simulink model "AFST_DD"  (R2016b)
settings: configuration reference "CodeGenConfigSet" (kept outside this file)
values from neighbouring files (symbols this model uses):
  Air_bDtyOrUType_C = Calibration.Parameter    [init_AFST_DD.m]    (also in init_AFST_DD_SIL.m = Simulink.Parameter)
  Air_facPerCorTAFS_C = Calibration.Parameter    [init_AFST_DD.m]    (also in init_AFST_DD_SIL.m = Simulink.Parameter)
  Air_rDtyCycMaxTAFS_C = Calibration.Parameter    [init_AFST_DD.m]    (also in init_AFST_DD_SIL.m = Simulink.Parameter)
  Air_rDtyCycMinTAFS_C = Calibration.Parameter    [init_AFST_DD.m]    (also in init_AFST_DD_SIL.m = Simulink.Parameter)
  Air_swtOscSelTAFS_C = Calibration.Parameter    [init_AFST_DD.m]    (also in init_AFST_DD_SIL.m = Simulink.Parameter)
  Air_tiDtyCycHiTAFSDefDeb_C = Calibration.Parameter    [init_AFST_DD.m]    (also in init_AFST_DD_SIL.m = Simulink.Parameter)
  Air_tiDtyCycHiTAFSOKDeb_C = Calibration.Parameter    [init_AFST_DD.m]    (also in init_AFST_DD_SIL.m = Simulink.Parameter)
  Air_tiDtyCycLoTAFSDefDeb_C = Calibration.Parameter    [init_AFST_DD.m]    (also in init_AFST_DD_SIL.m = Simulink.Parameter)
  Air_tiDtyCycLoTAFSOKDeb_C = Calibration.Parameter    [init_AFST_DD.m]    (also in init_AFST_DD_SIL.m = Simulink.Parameter)
  Air_tiPerHiTAFSDefDeb_C = Calibration.Parameter    [init_AFST_DD.m]    (also in init_AFST_DD_SIL.m = Simulink.Parameter)
  Air_tiPerHiTAFSOKDeb_C = Calibration.Parameter    [init_AFST_DD.m]    (also in init_AFST_DD_SIL.m = Simulink.Parameter)
  Air_tiPerLoTAFSDefDeb_C = Calibration.Parameter    [init_AFST_DD.m]    (also in init_AFST_DD_SIL.m = Simulink.Parameter)
  Air_tiPerLoTAFSOKDeb_C = Calibration.Parameter    [init_AFST_DD.m]    (also in init_AFST_DD_SIL.m = Simulink.Parameter)
  Air_tiPerRefTAFS_C = Calibration.Parameter    [init_AFST_DD.m]    (also in init_AFST_DD_SIL.m = Simulink.Parameter)
  Air_tiRefSigPerMaxTAFS_C = Calibration.Parameter    [init_AFST_DD.m]    (also in init_AFST_DD_SIL.m = Simulink.Parameter)
  Air_tiRefSigPerMinTAFS_C = Calibration.Parameter    [init_AFST_DD.m]    (also in init_AFST_DD_SIL.m = Simulink.Parameter)
  Air_tiVoltHiTAFSDefDeb_C = Calibration.Parameter    [init_AFST_DD.m]    (also in init_AFST_DD_SIL.m = Simulink.Parameter)
  Air_tiVoltHiTAFSOKDeb_C = Calibration.Parameter    [init_AFST_DD.m]    (also in init_AFST_DD_SIL.m = Simulink.Parameter)
  Air_tiVoltLoTAFSDefDeb_C = Calibration.Parameter    [init_AFST_DD.m]    (also in init_AFST_DD_SIL.m = Simulink.Parameter)
  Air_tiVoltLoTAFSOKDeb_C = Calibration.Parameter    [init_AFST_DD.m]    (also in init_AFST_DD_SIL.m = Simulink.Parameter)
  Air_tTransfTAFS_CUR = Calibration.Parameter    [init_AFST_DD.m]    (also in init_AFST_DD_SIL.m = Simulink.Parameter)
  Air_tTransfTAFS_CURX = Calibration.Parameter    [init_AFST_DD.m]    (also in init_AFST_DD_SIL.m = Simulink.Parameter)
  Air_utTransfTAFS_CUR = Calibration.Parameter    [init_AFST_DD.m]    (also in init_AFST_DD_SIL.m = Simulink.Parameter)
  Air_utTransfTAFS_CURX = Calibration.Parameter    [init_AFST_DD.m]    (also in init_AFST_DD_SIL.m = Simulink.Parameter)
  Air_uVoltMaxTAFS_C = Calibration.Parameter    [init_AFST_DD.m]    (also in init_AFST_DD_SIL.m = Simulink.Parameter)
  Air_uVoltMinTAFS_C = Calibration.Parameter    [init_AFST_DD.m]    (also in init_AFST_DD_SIL.m = Simulink.Parameter)
undefined symbols (not defined in the file or in its folder): AFST_DD_DT, Switch_conv
libraries: CXLib x18
settings Model: Creator=Colin  LastModifiedBy=guanxiaoxing
settings ConfigSetRef: SourceLocation=Base Workspace

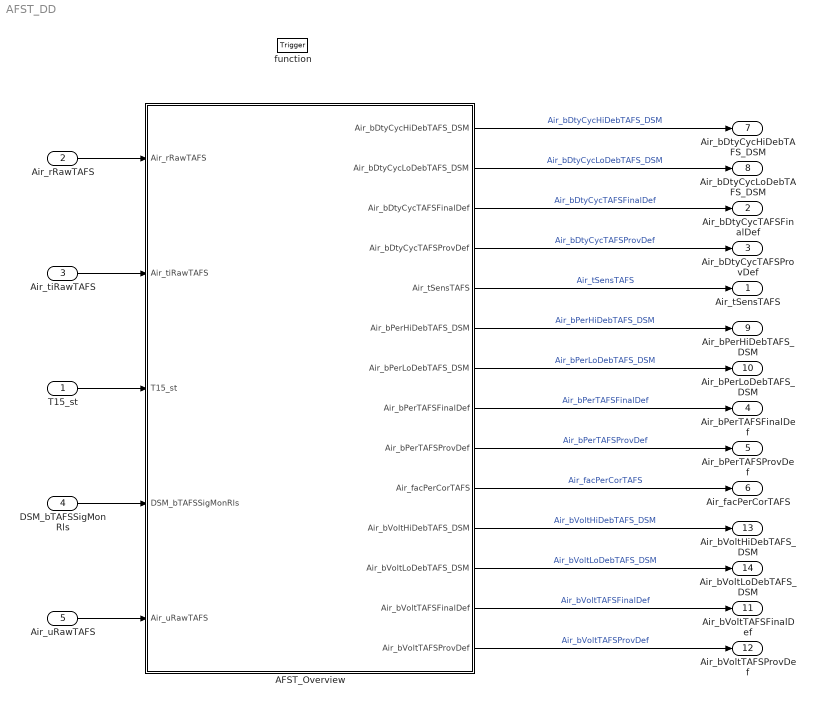
== system AFST_DD ==
  T15_st : Inport  Description=Terminal 15 status after debouncing  OutDataTypeStr=Enum: Switch_conv
  Air_rRawTAFS : Inport  Tag=%  Description=Duty cycle value of PWM signal from the temperature sensor at HFM position  Port=2  OutMin=0  OutMax=100  OutDataTypeStr=DutyCycle_rate
  Air_tiRawTAFS : Inport  Tag=ms  Description=Raw value of input time period of the temperature signal from HFM sensor  Port=3  OutMin=-107373  OutMax=107374  OutDataTypeStr=Time_Period_HFM6
  DSM_bTAFSSigMonRls : Inport  Description=fault flag of TAFS Signal Monitor  Port=4  OutMin=0  OutMax=1  OutDataTypeStr=boolean
  Air_uRawTAFS : Inport  Tag=mv  Description="Raw voltage value  from the temperature sensor at HFM position"  Port=5  OutMin=0  OutMax=5000  OutDataTypeStr=Ad_mv
  function : TriggerPort  TriggerType=function-call  VariantControl=Variant
  AFST_Overview : Subsystem
  Air_tSensTAFS : Outport  Tag=deg  Description=Sensed value of the air temperature at HFM position  OutMin=-200  OutMax=200  OutDataTypeStr=Temp_deg
  Air_bDtyCycTAFSFinalDef : Outport  Description=Fault flag of TAFS Duty Cycle Final fault  Port=2  OutMin=0  OutMax=1  OutDataTypeStr=boolean
  Air_bDtyCycTAFSProvDef : Outport  Description=Fault flag of TAFS Duty Cycle fault Proving  Port=3  OutMin=0  OutMax=1  OutDataTypeStr=boolean
  Air_bPerTAFSFinalDef : Outport  Description=Fault flag of TAFS Period Final fault  Port=4  OutMin=0  OutMax=1  OutDataTypeStr=boolean
  Air_bPerTAFSProvDef : Outport  Description=Fault flag of TAFS Period fault Proving  Port=5  OutMin=0  OutMax=1  OutDataTypeStr=boolean
  Air_facPerCorTAFS : Outport  Description=Period correction factor for air mass signal.  Port=6  OutMin=-4  OutMax=3.9999  OutDataTypeStr=Fact8192
  Air_bDtyCycHiDebTAFS_DSM : Outport  Description=Debounced fault of TAFS Duty Cycle High  Port=7  OutMin=0  OutMax=1  OutDataTypeStr=boolean
  Air_bDtyCycLoDebTAFS_DSM : Outport  Description=Debounced fault of TAFS Duty Cycle Low  Port=8  OutMin=0  OutMax=1  OutDataTypeStr=boolean
  Air_bPerHiDebTAFS_DSM : Outport  Description=Debounced fault of TAFS Period High  Port=9  OutMin=0  OutMax=1  OutDataTypeStr=boolean
  Air_bPerLoDebTAFS_DSM : Outport  Description=Debounced fault of TAFS Period Low  Port=10  OutMin=0  OutMax=1  OutDataTypeStr=boolean
  Air_bVoltTAFSFinalDef : Outport  Description=Fault flag of TAFS voltage Final fault  Port=11  OutMin=0  OutMax=1  OutDataTypeStr=boolean
  Air_bVoltTAFSProvDef : Outport  Description=Fault flag of TAFS voltage fault Proving  Port=12  OutMin=0  OutMax=1  OutDataTypeStr=boolean
  Air_bVoltHiDebTAFS_DSM : Outport  Description=Debounced fault of TAFS voltage High  Port=13  OutMin=0  OutMax=1  OutDataTypeStr=boolean
  Air_bVoltLoDebTAFS_DSM : Outport  Description="Debounced fault of TAFS  voltage Low"  Port=14  OutMin=0  OutMax=1  OutDataTypeStr=boolean
  wires:
  AFST_Overview/1(Air_bDtyCycHiDebTAFS_DSM) -> Air_bDtyCycHiDebTAFS_DSM/1  "Air_bDtyCycHiDebTAFS_DSM"
  AFST_Overview/3(Air_bDtyCycTAFSFinalDef) -> Air_bDtyCycTAFSFinalDef/1  "Air_bDtyCycTAFSFinalDef"
  AFST_Overview/4(Air_bDtyCycTAFSProvDef) -> Air_bDtyCycTAFSProvDef/1  "Air_bDtyCycTAFSProvDef"
  AFST_Overview/5(Air_tSensTAFS) -> Air_tSensTAFS/1  "Air_tSensTAFS"
  AFST_Overview/6(Air_bPerHiDebTAFS_DSM) -> Air_bPerHiDebTAFS_DSM/1  "Air_bPerHiDebTAFS_DSM"
  AFST_Overview/7(Air_bPerLoDebTAFS_DSM) -> Air_bPerLoDebTAFS_DSM/1  "Air_bPerLoDebTAFS_DSM"
  AFST_Overview/9(Air_bPerTAFSProvDef) -> Air_bPerTAFSProvDef/1  "Air_bPerTAFSProvDef"
  AFST_Overview/10(Air_facPerCorTAFS) -> Air_facPerCorTAFS/1  "Air_facPerCorTAFS"
  AFST_Overview/14(Air_bVoltTAFSProvDef) -> Air_bVoltTAFSProvDef/1  "Air_bVoltTAFSProvDef"
  AFST_Overview/11(Air_bVoltHiDebTAFS_DSM) -> Air_bVoltHiDebTAFS_DSM/1  "Air_bVoltHiDebTAFS_DSM"
  AFST_Overview/12(Air_bVoltLoDebTAFS_DSM) -> Air_bVoltLoDebTAFS_DSM/1  "Air_bVoltLoDebTAFS_DSM"
  AFST_Overview/2(Air_bDtyCycLoDebTAFS_DSM) -> Air_bDtyCycLoDebTAFS_DSM/1  "Air_bDtyCycLoDebTAFS_DSM"
  AFST_Overview/8(Air_bPerTAFSFinalDef) -> Air_bPerTAFSFinalDef/1  "Air_bPerTAFSFinalDef"
  AFST_Overview/13(Air_bVoltTAFSFinalDef) -> Air_bVoltTAFSFinalDef/1  "Air_bVoltTAFSFinalDef"
  Air_rRawTAFS/1 -> AFST_Overview/1(Air_rRawTAFS)
  Air_tiRawTAFS/1 -> AFST_Overview/2(Air_tiRawTAFS)
  T15_st/1 -> AFST_Overview/3(T15_st)
  DSM_bTAFSSigMonRls/1 -> AFST_Overview/4(DSM_bTAFSSigMonRls)
  Air_uRawTAFS/1 -> AFST_Overview/5(Air_uRawTAFS)

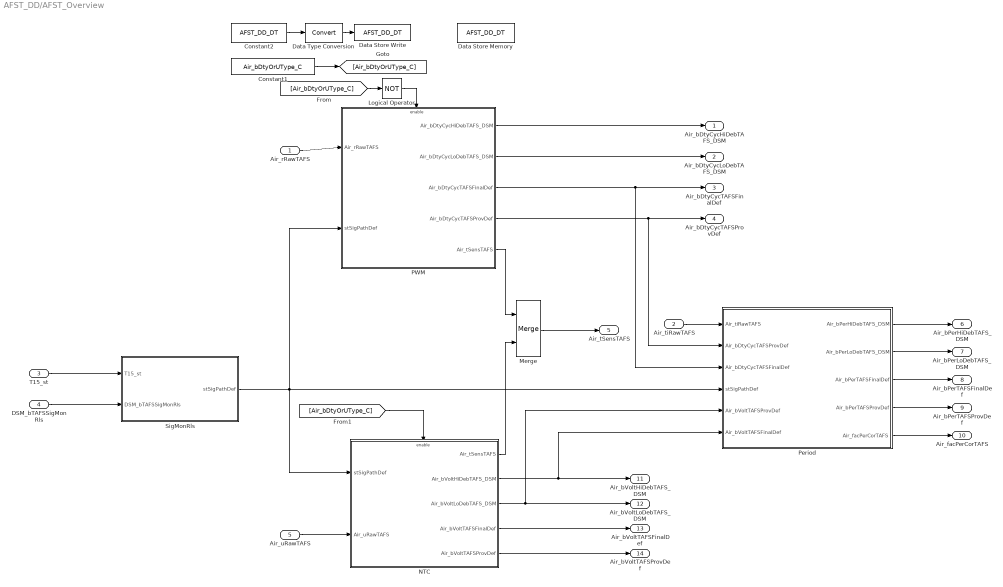
== system AFST_DD/AFST_Overview ==
  Air_rRawTAFS : Inport
  Air_tiRawTAFS : Inport  Port=2
  T15_st : Inport  Port=3
  DSM_bTAFSSigMonRls : Inport  Port=4
  Air_uRawTAFS : Inport  Port=5
  Constant1 : Constant  Value=Air_bDtyOrUType_C
  Constant2 : Constant  Value=AFST_DD_DT
  Data Store Memory : DataStoreMemory  DataStoreName=AFST_DD_DT  ReadBeforeWriteMsg=warning  WriteAfterWriteMsg=warning  WriteAfterReadMsg=warning  ShowAdditionalParam=off
  Data Store Write : DataStoreWrite  DataStoreName=AFST_DD_DT
  Data Type Conversion : DataTypeConversion
  Logical Operator : Logic  Operator=NOT  AllPortsSameDT=off  OutDataTypeStr=boolean
  Merge : Merge
  NTC : Subsystem
  PWM : Subsystem
  Period : Subsystem
  SigMonRls : Subsystem
  Air_bDtyCycHiDebTAFS_DSM : Outport
  Air_bDtyCycLoDebTAFS_DSM : Outport  Port=2
  Air_bDtyCycTAFSFinalDef : Outport  Port=3
  Air_bDtyCycTAFSProvDef : Outport  Port=4
  Air_tSensTAFS : Outport  Port=5
  Air_bPerHiDebTAFS_DSM : Outport  Port=6
  Air_bPerLoDebTAFS_DSM : Outport  Port=7
  Air_bPerTAFSFinalDef : Outport  Port=8
  Air_bPerTAFSProvDef : Outport  Port=9
  Air_facPerCorTAFS : Outport  Port=10
  Air_bVoltHiDebTAFS_DSM : Outport  Port=11
  Air_bVoltLoDebTAFS_DSM : Outport  Port=12
  Air_bVoltTAFSFinalDef : Outport  Port=13
  Air_bVoltTAFSProvDef : Outport  Port=14
  wires:
  NTC/3(Air_bVoltLoDebTAFS_DSM) -> Air_bVoltLoDebTAFS_DSM/1, Period/5(Air_bVoltTAFSProvDef)
  Period/4(Air_bPerTAFSProvDef) -> Air_bPerTAFSProvDef/1
  PWM/3(Air_bDtyCycTAFSFinalDef) -> Air_bDtyCycTAFSFinalDef/1, Period/3(Air_bDtyCycTAFSFinalDef)
  PWM/2(Air_bDtyCycLoDebTAFS_DSM) -> Air_bDtyCycLoDebTAFS_DSM/1
  NTC/4(Air_bVoltTAFSFinalDef) -> Air_bVoltTAFSFinalDef/1
  PWM/4(Air_bDtyCycTAFSProvDef) -> Air_bDtyCycTAFSProvDef/1, Period/2(Air_bDtyCycTAFSProvDef)
  DSM_bTAFSSigMonRls/1 -> SigMonRls/2(DSM_bTAFSSigMonRls)
  Constant2/1 -> Data Type Conversion/1
  Air_uRawTAFS/1 -> NTC/2(Air_uRawTAFS)
  Period/1(Air_bPerHiDebTAFS_DSM) -> Air_bPerHiDebTAFS_DSM/1
  NTC/5(Air_bVoltTAFSProvDef) -> Air_bVoltTAFSProvDef/1
  Merge/1 -> Air_tSensTAFS/1
  PWM/5(Air_tSensTAFS) -> Merge/1
  NTC/1(Air_tSensTAFS) -> Merge/2
  Air_rRawTAFS/1 -> PWM/1(Air_rRawTAFS)
  PWM/1(Air_bDtyCycHiDebTAFS_DSM) -> Air_bDtyCycHiDebTAFS_DSM/1
  [Air_bDtyOrUType_C] -> NTC/Enable
  Period/2(Air_bPerLoDebTAFS_DSM) -> Air_bPerLoDebTAFS_DSM/1
  Constant1/1 -> [Air_bDtyOrUType_C]
  T15_st/1 -> SigMonRls/1(T15_st)
  SigMonRls/1(stSigPathDef) -> PWM/2(stSigPathDef), Period/4(stSigPathDef), NTC/1(stSigPathDef)
  [Air_bDtyOrUType_C] -> Logical Operator/1
  Logical Operator/1 -> PWM/Enable
  Air_tiRawTAFS/1 -> Period/1(Air_tiRawTAFS)
  Data Type Conversion/1 -> Data Store Write/1
  NTC/2(Air_bVoltHiDebTAFS_DSM) -> Air_bVoltHiDebTAFS_DSM/1, Period/6(Air_bVoltTAFSFinalDef)
  Period/5(Air_facPerCorTAFS) -> Air_facPerCorTAFS/1
  Period/3(Air_bPerTAFSFinalDef) -> Air_bPerTAFSFinalDef/1

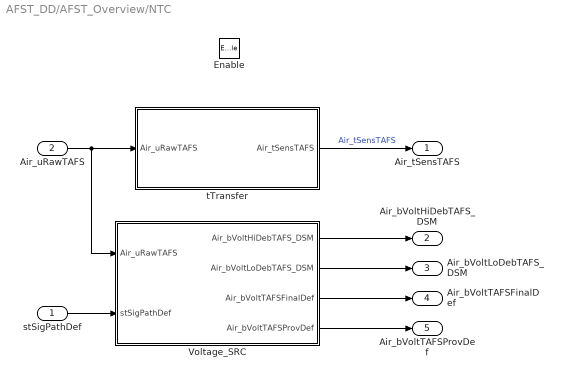
== system AFST_DD/AFST_Overview/NTC ==
  stSigPathDef : Inport
  Air_uRawTAFS : Inport  Port=2
  Enable : EnablePort
  Voltage_SRC : Subsystem
  tTransfer : Subsystem
  Air_tSensTAFS : Outport
  Air_bVoltHiDebTAFS_DSM : Outport  Port=2
  Air_bVoltLoDebTAFS_DSM : Outport  Port=3
  Air_bVoltTAFSFinalDef : Outport  Port=4
  Air_bVoltTAFSProvDef : Outport  Port=5
  wires:
  stSigPathDef/1 -> Voltage_SRC/2(stSigPathDef)
  Air_uRawTAFS/1 -> Voltage_SRC/1(Air_uRawTAFS), tTransfer/1(Air_uRawTAFS)
  tTransfer/1(Air_tSensTAFS) -> Air_tSensTAFS/1  "Air_tSensTAFS"
  Voltage_SRC/1(Air_bVoltHiDebTAFS_DSM) -> Air_bVoltHiDebTAFS_DSM/1
  Voltage_SRC/2(Air_bVoltLoDebTAFS_DSM) -> Air_bVoltLoDebTAFS_DSM/1
  Voltage_SRC/3(Air_bVoltTAFSFinalDef) -> Air_bVoltTAFSFinalDef/1
  Voltage_SRC/4(Air_bVoltTAFSProvDef) -> Air_bVoltTAFSProvDef/1

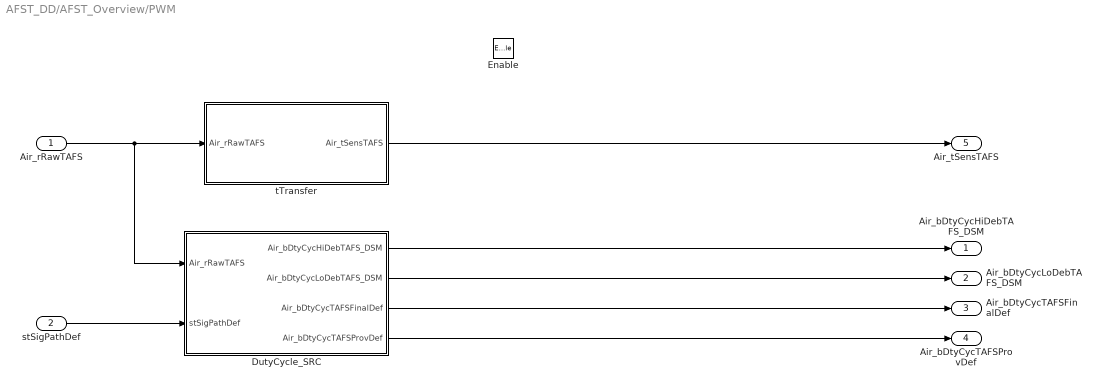
== system AFST_DD/AFST_Overview/PWM ==
  Air_rRawTAFS : Inport
  stSigPathDef : Inport  Port=2
  Enable : EnablePort
  "DutyCycle_SRC " : Subsystem
  tTransfer : Subsystem
  Air_bDtyCycHiDebTAFS_DSM : Outport
  Air_bDtyCycLoDebTAFS_DSM : Outport  Port=2
  Air_bDtyCycTAFSFinalDef : Outport  Port=3
  Air_bDtyCycTAFSProvDef : Outport  Port=4
  Air_tSensTAFS : Outport  Port=5
  wires:
  Air_rRawTAFS/1 -> tTransfer/1(Air_rRawTAFS), "DutyCycle_SRC "/1(Air_rRawTAFS)
  "DutyCycle_SRC "/3(Air_bDtyCycTAFSFinalDef) -> Air_bDtyCycTAFSFinalDef/1
  stSigPathDef/1 -> "DutyCycle_SRC "/2(stSigPathDef)
  "DutyCycle_SRC "/2(Air_bDtyCycLoDebTAFS_DSM) -> Air_bDtyCycLoDebTAFS_DSM/1
  "DutyCycle_SRC "/4(Air_bDtyCycTAFSProvDef) -> Air_bDtyCycTAFSProvDef/1
  "DutyCycle_SRC "/1(Air_bDtyCycHiDebTAFS_DSM) -> Air_bDtyCycHiDebTAFS_DSM/1
  tTransfer/1(Air_tSensTAFS) -> Air_tSensTAFS/1

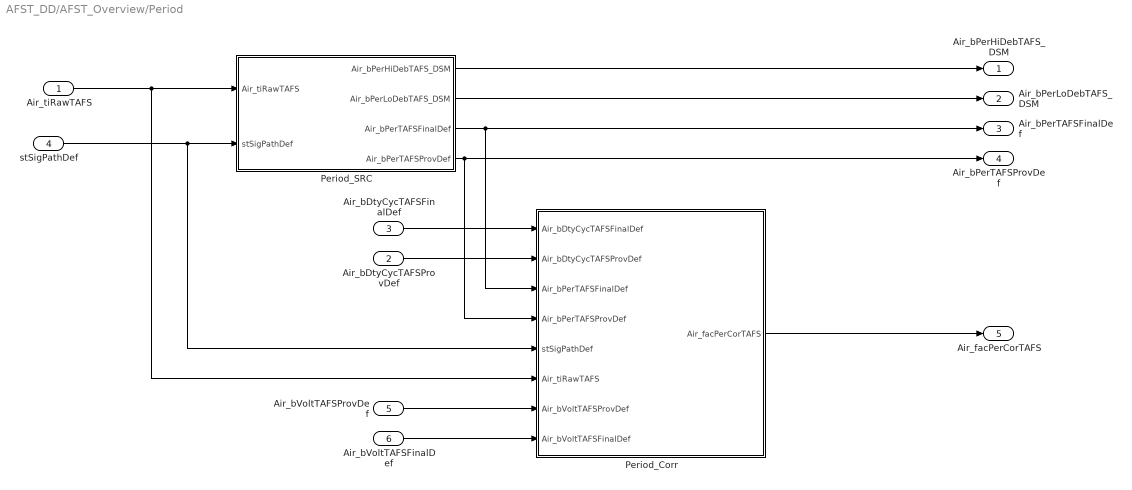
== system AFST_DD/AFST_Overview/Period ==
  Air_tiRawTAFS : Inport
  Air_bDtyCycTAFSProvDef : Inport  Port=2
  Air_bDtyCycTAFSFinalDef : Inport  Port=3
  stSigPathDef : Inport  Port=4
  Air_bVoltTAFSProvDef : Inport  Port=5
  Air_bVoltTAFSFinalDef : Inport  Port=6
  Period_Corr : Subsystem
  Period_SRC : Subsystem
  Air_bPerHiDebTAFS_DSM : Outport
  Air_bPerLoDebTAFS_DSM : Outport  Port=2
  Air_bPerTAFSFinalDef : Outport  Port=3
  Air_bPerTAFSProvDef : Outport  Port=4
  Air_facPerCorTAFS : Outport  Port=5
  wires:
  Air_tiRawTAFS/1 -> Period_SRC/1(Air_tiRawTAFS), Period_Corr/6(Air_tiRawTAFS)
  Period_SRC/4(Air_bPerTAFSProvDef) -> Air_bPerTAFSProvDef/1, Period_Corr/4(Air_bPerTAFSProvDef)
  Period_Corr/1(Air_facPerCorTAFS) -> Air_facPerCorTAFS/1
  Period_SRC/3(Air_bPerTAFSFinalDef) -> Air_bPerTAFSFinalDef/1, Period_Corr/3(Air_bPerTAFSFinalDef)
  Period_SRC/2(Air_bPerLoDebTAFS_DSM) -> Air_bPerLoDebTAFS_DSM/1
  Period_SRC/1(Air_bPerHiDebTAFS_DSM) -> Air_bPerHiDebTAFS_DSM/1
  Air_bDtyCycTAFSProvDef/1 -> Period_Corr/2(Air_bDtyCycTAFSProvDef)
  Air_bDtyCycTAFSFinalDef/1 -> Period_Corr/1(Air_bDtyCycTAFSFinalDef)
  stSigPathDef/1 -> Period_SRC/2(stSigPathDef), Period_Corr/5(stSigPathDef)
  Air_bVoltTAFSFinalDef/1 -> Period_Corr/8(Air_bVoltTAFSFinalDef)
  Air_bVoltTAFSProvDef/1 -> Period_Corr/7(Air_bVoltTAFSProvDef)

== system AFST_DD/AFST_Overview/SigMonRls ==
  T15_st : Inport
  DSM_bTAFSSigMonRls : Inport  Port=2
  Constant : Constant  Value=Switch_conv.ON
  Logical Operator : Logic  AllPortsSameDT=off  OutDataTypeStr=boolean
  Relational Operator : RelationalOperator  Operator===  OutDataTypeStr=boolean  RndMeth=Simplest
  stSigPathDef : Outport
  wires:
  T15_st/1 -> Relational Operator/1
  Logical Operator/1 -> stSigPathDef/1
  Relational Operator/1 -> Logical Operator/1
  DSM_bTAFSSigMonRls/1 -> Logical Operator/2
  Constant/1 -> Relational Operator/2

== system AFST_DD/AFST_Overview/NTC/Voltage_SRC ==
  Air_uRawTAFS : Inport
  stSigPathDef : Inport  Port=2
  FinalDef : Subsystem
  ProvDef : Subsystem
  SRCHi : Subsystem
  SRCLo : Subsystem
  Air_bVoltHiDebTAFS_DSM : Outport
  Air_bVoltLoDebTAFS_DSM : Outport  Port=2
  Air_bVoltTAFSFinalDef : Outport  Port=3
  Air_bVoltTAFSProvDef : Outport  Port=4
  wires:
  Air_uRawTAFS/1 -> SRCLo/1(Air_uRawTAFS), SRCHi/1(Air_uRawTAFS)
  SRCHi/1(Air_bVoltHiDebTAFS_DSM) -> FinalDef/1(Air_bVoltHiDebTAFS_DSM), Air_bVoltHiDebTAFS_DSM/1
  SRCLo/1(Air_bVoltLoDebTAFS_DSM) -> Air_bVoltLoDebTAFS_DSM/1, FinalDef/2(Air_bVoltLoDebTAFS_DSM)
  stSigPathDef/1 -> SRCHi/2(stSigPathDef), SRCLo/2(stSigPathDef), FinalDef/3(stSigPathDef)
  SRCLo/2(bVoltLo) -> ProvDef/3(bVoltLo)
  SRCHi/2(bVoltHi) -> ProvDef/2(bVoltHi)
  FinalDef/1(Air_bVoltTAFSFinalDef) -> Air_bVoltTAFSFinalDef/1, ProvDef/1(Air_bVoltTAFSFinalDef)
  ProvDef/1(Air_bVoltTAFSProvDef) -> Air_bVoltTAFSProvDef/1

== system AFST_DD/AFST_Overview/NTC/tTransfer ==
  Air_uRawTAFS : Inport
  Air_utTransfTAFS_CUR : Lookup_n-D  NumberOfTableDimensions=1  BreakpointsForDimension1=Air_utTransfTAFS_CURX  BreakpointsForDimension2=[1:3]  IndexSearchMethod=Linear search  BeginIndexSearchUsingPreviousIndexResult=on  Table=Air_utTransfTAFS_CUR  TableDataTypeStr=Inherit: Inherit from 'Table data'  ExtrapMethod=Clip  InternalRulePriority=Speed  OutDataTypeStr=Inherit: Inherit from 'Table data'  RndMeth=Simplest  InputSameDT=on
  Air_tSensTAFS : Outport
  wires:
  Air_uRawTAFS/1 -> Air_utTransfTAFS_CUR/1
  Air_utTransfTAFS_CUR/1 -> Air_tSensTAFS/1

== system AFST_DD/AFST_Overview/PWM/DutyCycle_SRC  ==
  Air_rRawTAFS : Inport
  stSigPathDef : Inport  Port=2
  FinalDef : Subsystem
  ProvDef : Subsystem
  SRCHi : Subsystem
  SRCLo : Subsystem
  Air_bDtyCycHiDebTAFS_DSM : Outport
  Air_bDtyCycLoDebTAFS_DSM : Outport  Port=2
  Air_bDtyCycTAFSFinalDef : Outport  Port=3
  Air_bDtyCycTAFSProvDef : Outport  Port=4
  wires:
  Air_rRawTAFS/1 -> SRCLo/1(Air_rRawTAFS), SRCHi/1(Air_rRawTAFS)
  SRCHi/1(Air_bDtyCycHiDebTAFS_DSM) -> FinalDef/1(Air_bDtyCycHiDebTAFS_DSM), Air_bDtyCycHiDebTAFS_DSM/1
  SRCLo/1(Air_bDtyCycLoDebTAFS_DSM) -> Air_bDtyCycLoDebTAFS_DSM/1, FinalDef/2(Air_bDtyCycLoDebTAFS_DSM)
  stSigPathDef/1 -> SRCHi/2(stSigPathDef), SRCLo/2(stSigPathDef), FinalDef/3(stSigPathDef)
  SRCLo/2(bDtyCycLo) -> ProvDef/3(bDtyCycLo)
  SRCHi/2(bDtyCycHi) -> ProvDef/2(bDtyCycHi)
  FinalDef/1(Air_bDtyCycTAFSFinalDef) -> Air_bDtyCycTAFSFinalDef/1, ProvDef/1(Air_bDtyCycTAFSFinalDef)
  ProvDef/1(Air_bDtyCycTAFSProvDef) -> Air_bDtyCycTAFSProvDef/1

== system AFST_DD/AFST_Overview/PWM/tTransfer ==
  Air_rRawTAFS : Inport
  Air_tTransfTAFS_CUR : Lookup_n-D  NumberOfTableDimensions=1  BreakpointsForDimension1=Air_tTransfTAFS_CURX  BreakpointsForDimension2=[1:3]  IndexSearchMethod=Linear search  BeginIndexSearchUsingPreviousIndexResult=on  Table=Air_tTransfTAFS_CUR  TableDataTypeStr=Inherit: Inherit from 'Table data'  ExtrapMethod=Clip  InternalRulePriority=Speed  OutDataTypeStr=Inherit: Inherit from 'Table data'  RndMeth=Simplest  InputSameDT=on
  Air_tSensTAFS : Outport
  wires:
  Air_rRawTAFS/1 -> Air_tTransfTAFS_CUR/1
  Air_tTransfTAFS_CUR/1 -> Air_tSensTAFS/1

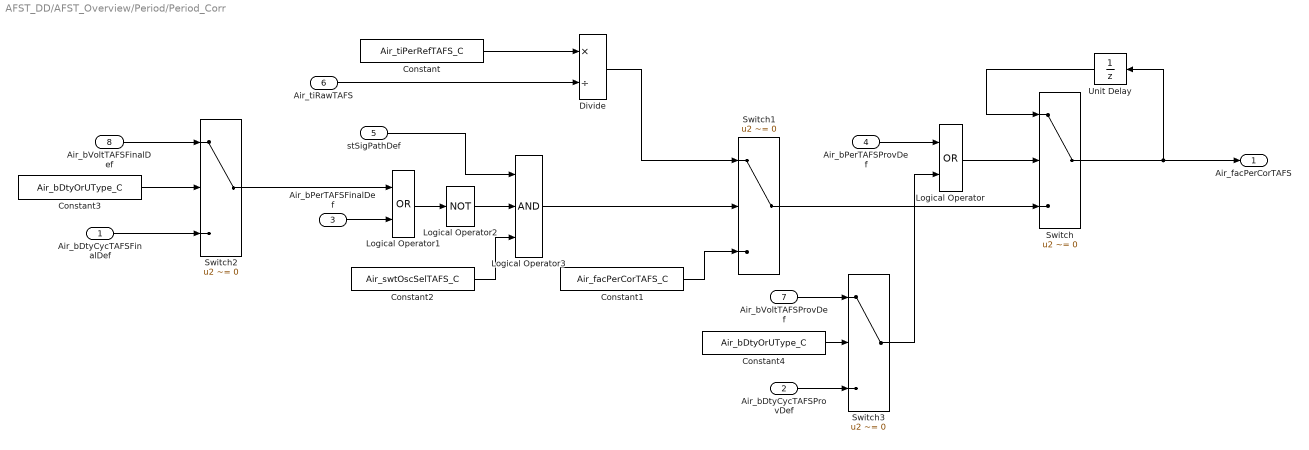
== system AFST_DD/AFST_Overview/Period/Period_Corr ==
  Air_bDtyCycTAFSFinalDef : Inport
  Air_bDtyCycTAFSProvDef : Inport  Port=2
  Air_bPerTAFSFinalDef : Inport  Port=3
  Air_bPerTAFSProvDef : Inport  Port=4
  stSigPathDef : Inport  Port=5
  Air_tiRawTAFS : Inport  Port=6
  Air_bVoltTAFSProvDef : Inport  Port=7
  Air_bVoltTAFSFinalDef : Inport  Port=8
  Constant : Constant  Value=Air_tiPerRefTAFS_C
  Constant1 : Constant  Value=Air_facPerCorTAFS_C
  Constant2 : Constant  Value=Air_swtOscSelTAFS_C
  Constant3 : Constant  Value=Air_bDtyOrUType_C
  Constant4 : Constant  Value=Air_bDtyOrUType_C
  Divide : Product  Inputs=*/  OutDataTypeStr=Inherit: Inherit via back propagation
  Logical Operator : Logic  Operator=OR  AllPortsSameDT=off  OutDataTypeStr=boolean
  Logical Operator1 : Logic  Operator=OR  AllPortsSameDT=off  OutDataTypeStr=boolean
  Logical Operator2 : Logic  Operator=NOT  AllPortsSameDT=off  OutDataTypeStr=boolean
  Logical Operator3 : Logic  Inputs=3  AllPortsSameDT=off  OutDataTypeStr=boolean
  Switch : Switch  Criteria=u2 ~= 0  OutDataTypeStr=Inherit: Inherit via back propagation
  Switch1 : Switch  Criteria=u2 ~= 0  OutDataTypeStr=Inherit: Inherit via back propagation  InputSameDT=on
  Switch2 : Switch  Criteria=u2 ~= 0  OutDataTypeStr=Inherit: Inherit via back propagation  InputSameDT=on
  Switch3 : Switch  Criteria=u2 ~= 0  OutDataTypeStr=Inherit: Inherit via back propagation  InputSameDT=on
  Unit Delay : UnitDelay  InitialCondition=1  SampleTime=-1
      settings: AttributesFormatString=InitialValue=%<InitialCondition>
  Air_facPerCorTAFS : Outport
  wires:
  Switch/1 -> Unit Delay/1, Air_facPerCorTAFS/1
  Unit Delay/1 -> Switch/1
  Air_bPerTAFSProvDef/1 -> Logical Operator/1
  Logical Operator/1 -> Switch/2
  Switch1/1 -> Switch/3
  Constant1/1 -> Switch1/3
  Constant/1 -> Divide/1
  Air_tiRawTAFS/1 -> Divide/2
  Divide/1 -> Switch1/1
  Switch2/1 -> Logical Operator1/1
  Air_bPerTAFSFinalDef/1 -> Logical Operator1/2
  Logical Operator1/1 -> Logical Operator2/1
  stSigPathDef/1 -> Logical Operator3/1
  Logical Operator2/1 -> Logical Operator3/2
  Constant2/1 -> Logical Operator3/3
  Logical Operator3/1 -> Switch1/2
  Constant3/1 -> Switch2/2
  Air_bDtyCycTAFSFinalDef/1 -> Switch2/3
  Air_bVoltTAFSFinalDef/1 -> Switch2/1
  Constant4/1 -> Switch3/2
  Air_bVoltTAFSProvDef/1 -> Switch3/1
  Air_bDtyCycTAFSProvDef/1 -> Switch3/3
  Switch3/1 -> Logical Operator/2

== system AFST_DD/AFST_Overview/Period/Period_SRC ==
  Air_tiRawTAFS : Inport
  stSigPathDef : Inport  Port=2
  FinalDef : Subsystem
  ProvDef : Subsystem
  SRCHi : Subsystem
  SRCLo : Subsystem
  Air_bPerHiDebTAFS_DSM : Outport
  Air_bPerLoDebTAFS_DSM : Outport  Port=2
  Air_bPerTAFSFinalDef : Outport  Port=3
  Air_bPerTAFSProvDef : Outport  Port=4
  wires:
  Air_tiRawTAFS/1 -> SRCLo/1(Air_tiRawTAFS), SRCHi/1(Air_tiRawTAFS)
  SRCHi/1(Air_bPerHiDebTAFS_DSM) -> FinalDef/1(Air_bPerHiDebTAFS_DSM), Air_bPerHiDebTAFS_DSM/1
  SRCLo/1(Air_bPerLoDebTAFS_DSM) -> Air_bPerLoDebTAFS_DSM/1, FinalDef/2(Air_bPerLoDebTAFS_DSM)
  stSigPathDef/1 -> SRCHi/2(stSigPathDef), SRCLo/2(stSigPathDef), FinalDef/3(stSigPathDef)
  SRCLo/2(bDtyCycLo) -> ProvDef/3(bDtyCycLo)
  SRCHi/2(bDtyCycHi) -> ProvDef/2(bDtyCycHi)
  FinalDef/1(Air_bPerTAFSFinalDef) -> Air_bPerTAFSFinalDef/1, ProvDef/1(Air_bPerTAFSFinalDef)
  ProvDef/1(Air_bPerTAFSProvDef) -> Air_bPerTAFSProvDef/1

== system AFST_DD/AFST_Overview/NTC/Voltage_SRC/FinalDef ==
  Air_bVoltHiDebTAFS_DSM : Inport
  Air_bVoltLoDebTAFS_DSM : Inport  Port=2
  stSigPathDef : Inport  Port=3
  Logical Operator : Logic  Operator=NOT  AllPortsSameDT=off  OutDataTypeStr=boolean
  Logical Operator1 : Logic  Operator=OR  AllPortsSameDT=off  OutDataTypeStr=boolean
  Logical Operator6 : Logic  Operator=OR  AllPortsSameDT=off  OutDataTypeStr=boolean
  Air_bVoltTAFSFinalDef : Outport
  wires:
  Logical Operator6/1 -> Air_bVoltTAFSFinalDef/1
  Air_bVoltHiDebTAFS_DSM/1 -> Logical Operator1/1
  Air_bVoltLoDebTAFS_DSM/1 -> Logical Operator1/2
  Logical Operator1/1 -> Logical Operator6/1
  stSigPathDef/1 -> Logical Operator/1
  Logical Operator/1 -> Logical Operator6/2

== system AFST_DD/AFST_Overview/NTC/Voltage_SRC/ProvDef ==
  Air_bVoltTAFSFinalDef : Inport
  bVoltHi : Inport  Port=2
  bVoltLo : Inport  Port=3
  Logical Operator : Logic  Operator=OR  AllPortsSameDT=off  OutDataTypeStr=boolean
  Logical Operator1 : Logic  AllPortsSameDT=off  OutDataTypeStr=boolean
  Logical Operator2 : Logic  Operator=NOT  AllPortsSameDT=off  OutDataTypeStr=boolean
  Air_bVoltTAFSProvDef : Outport
  wires:
  bVoltHi/1 -> Logical Operator/1
  bVoltLo/1 -> Logical Operator/2
  Logical Operator/1 -> Logical Operator1/1
  Air_bVoltTAFSFinalDef/1 -> Logical Operator2/1
  Logical Operator2/1 -> Logical Operator1/2
  Logical Operator1/1 -> Air_bVoltTAFSProvDef/1

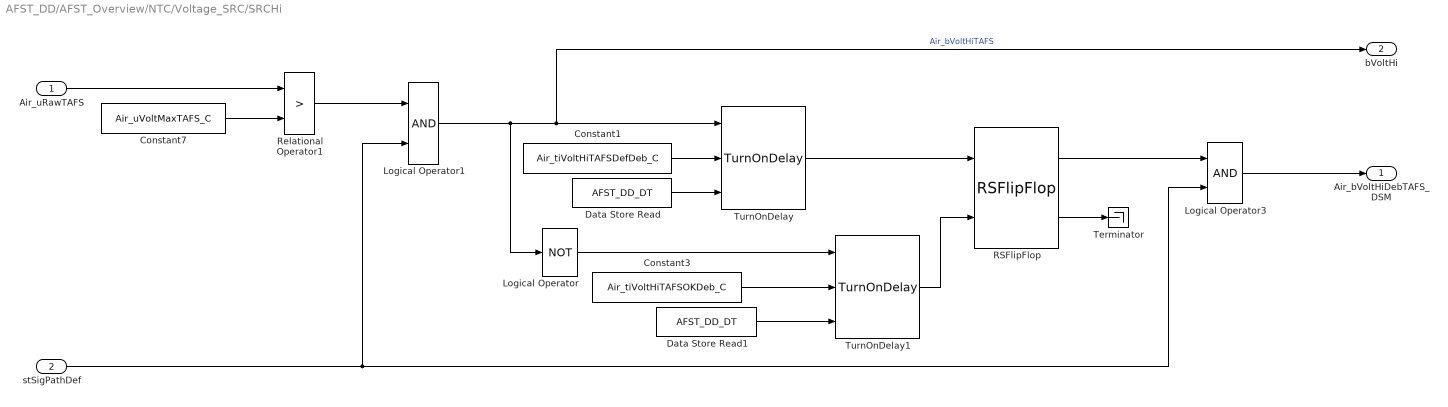
== system AFST_DD/AFST_Overview/NTC/Voltage_SRC/SRCHi ==
  Air_uRawTAFS : Inport
  stSigPathDef : Inport  Port=2
  Constant1 : Constant  Value=Air_tiVoltHiTAFSDefDeb_C
  Constant3 : Constant  Value=Air_tiVoltHiTAFSOKDeb_C
  Constant7 : Constant  Value=Air_uVoltMaxTAFS_C
  Data Store Read : DataStoreRead  DataStoreName=AFST_DD_DT
  Data Store Read1 : DataStoreRead  DataStoreName=AFST_DD_DT
  Logical Operator : Logic  Operator=NOT  AllPortsSameDT=off  OutDataTypeStr=boolean
  Logical Operator1 : Logic  AllPortsSameDT=off  OutDataTypeStr=boolean
  Logical Operator3 : Logic  AllPortsSameDT=off  OutDataTypeStr=boolean
  RSFlipFlop : CXLib/RSFlipFlop
  Relational Operator1 : RelationalOperator  Operator=>  OutDataTypeStr=boolean  RndMeth=Simplest
  Terminator : Terminator
  TurnOnDelay : CXLib/TurnOnDelay
  TurnOnDelay1 : CXLib/TurnOnDelay
  Air_bVoltHiDebTAFS_DSM : Outport
  bVoltHi : Outport  Port=2
  wires:
  Constant3/1 -> TurnOnDelay1/2
  Logical Operator1/1 -> Logical Operator/1, bVoltHi/1, TurnOnDelay/1  "Air_bVoltHiTAFS"
  Logical Operator/1 -> TurnOnDelay1/1
  Relational Operator1/1 -> Logical Operator1/1
  Constant7/1 -> Relational Operator1/2
  Data Store Read1/1 -> TurnOnDelay1/3
  Constant1/1 -> TurnOnDelay/2
  Data Store Read/1 -> TurnOnDelay/3
  RSFlipFlop/2 -> Terminator/1
  TurnOnDelay/1 -> RSFlipFlop/1
  TurnOnDelay1/1 -> RSFlipFlop/2
  Logical Operator3/1 -> Air_bVoltHiDebTAFS_DSM/1
  Air_uRawTAFS/1 -> Relational Operator1/1
  stSigPathDef/1 -> Logical Operator3/2, Logical Operator1/2
  RSFlipFlop/1 -> Logical Operator3/1

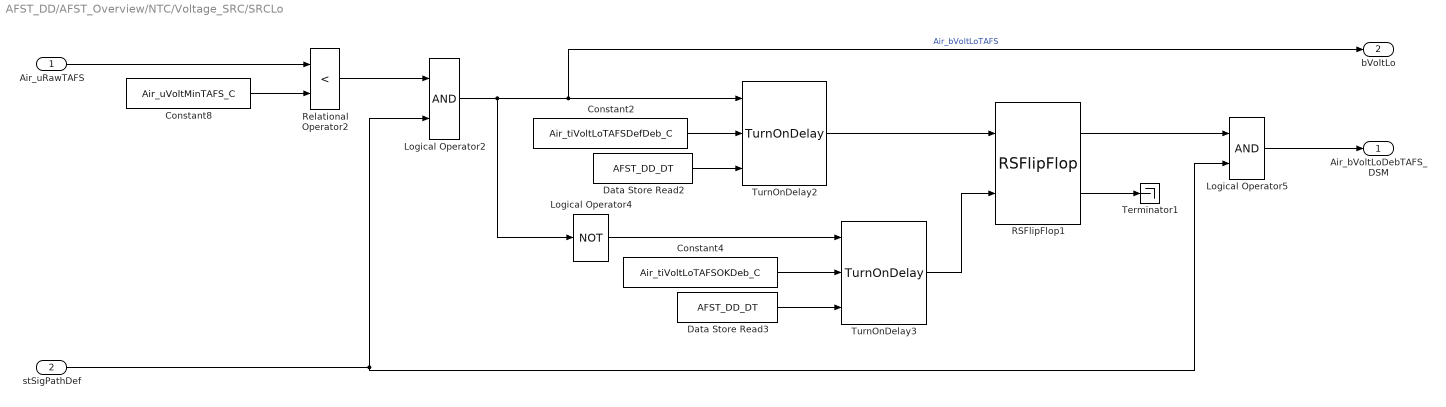
== system AFST_DD/AFST_Overview/NTC/Voltage_SRC/SRCLo ==
  Air_uRawTAFS : Inport
  stSigPathDef : Inport  Port=2
  Constant2 : Constant  Value=Air_tiVoltLoTAFSDefDeb_C
  Constant4 : Constant  Value=Air_tiVoltLoTAFSOKDeb_C
  Constant8 : Constant  Value=Air_uVoltMinTAFS_C
  Data Store Read2 : DataStoreRead  DataStoreName=AFST_DD_DT
  Data Store Read3 : DataStoreRead  DataStoreName=AFST_DD_DT
  Logical Operator2 : Logic  AllPortsSameDT=off  OutDataTypeStr=boolean
  Logical Operator4 : Logic  Operator=NOT  AllPortsSameDT=off  OutDataTypeStr=boolean
  Logical Operator5 : Logic  AllPortsSameDT=off  OutDataTypeStr=boolean
  RSFlipFlop1 : CXLib/RSFlipFlop
  Relational Operator2 : RelationalOperator  Operator=<  OutDataTypeStr=boolean  RndMeth=Simplest
  Terminator1 : Terminator
  TurnOnDelay2 : CXLib/TurnOnDelay
  TurnOnDelay3 : CXLib/TurnOnDelay
  Air_bVoltLoDebTAFS_DSM : Outport
  bVoltLo : Outport  Port=2
  wires:
  Data Store Read2/1 -> TurnOnDelay2/3
  Data Store Read3/1 -> TurnOnDelay3/3
  Constant8/1 -> Relational Operator2/2
  Relational Operator2/1 -> Logical Operator2/1
  Constant2/1 -> TurnOnDelay2/2
  Constant4/1 -> TurnOnDelay3/2
  Logical Operator4/1 -> TurnOnDelay3/1
  TurnOnDelay2/1 -> RSFlipFlop1/1
  RSFlipFlop1/1 -> Logical Operator5/1
  Logical Operator5/1 -> Air_bVoltLoDebTAFS_DSM/1
  RSFlipFlop1/2 -> Terminator1/1
  TurnOnDelay3/1 -> RSFlipFlop1/2
  stSigPathDef/1 -> Logical Operator5/2, Logical Operator2/2
  Logical Operator2/1 -> Logical Operator4/1, bVoltLo/1, TurnOnDelay2/1  "Air_bVoltLoTAFS"
  Air_uRawTAFS/1 -> Relational Operator2/1

== system AFST_DD/AFST_Overview/PWM/DutyCycle_SRC /FinalDef ==
  Air_bDtyCycHiDebTAFS_DSM : Inport
  Air_bDtyCycLoDebTAFS_DSM : Inport  Port=2
  stSigPathDef : Inport  Port=3
  Logical Operator : Logic  Operator=NOT  AllPortsSameDT=off  OutDataTypeStr=boolean
  Logical Operator1 : Logic  Operator=OR  AllPortsSameDT=off  OutDataTypeStr=boolean
  Logical Operator6 : Logic  Operator=OR  AllPortsSameDT=off  OutDataTypeStr=boolean
  Air_bDtyCycTAFSFinalDef : Outport
  wires:
  Logical Operator6/1 -> Air_bDtyCycTAFSFinalDef/1
  Air_bDtyCycHiDebTAFS_DSM/1 -> Logical Operator1/1
  Air_bDtyCycLoDebTAFS_DSM/1 -> Logical Operator1/2
  Logical Operator1/1 -> Logical Operator6/1
  stSigPathDef/1 -> Logical Operator/1
  Logical Operator/1 -> Logical Operator6/2

== system AFST_DD/AFST_Overview/PWM/DutyCycle_SRC /ProvDef ==
  Air_bDtyCycTAFSFinalDef : Inport
  bDtyCycHi : Inport  Port=2
  bDtyCycLo : Inport  Port=3
  Logical Operator : Logic  Operator=OR  AllPortsSameDT=off  OutDataTypeStr=boolean
  Logical Operator1 : Logic  AllPortsSameDT=off  OutDataTypeStr=boolean
  Logical Operator2 : Logic  Operator=NOT  AllPortsSameDT=off  OutDataTypeStr=boolean
  Air_bDtyCycTAFSProvDef : Outport
  wires:
  bDtyCycHi/1 -> Logical Operator/1
  bDtyCycLo/1 -> Logical Operator/2
  Logical Operator/1 -> Logical Operator1/1
  Air_bDtyCycTAFSFinalDef/1 -> Logical Operator2/1
  Logical Operator2/1 -> Logical Operator1/2
  Logical Operator1/1 -> Air_bDtyCycTAFSProvDef/1

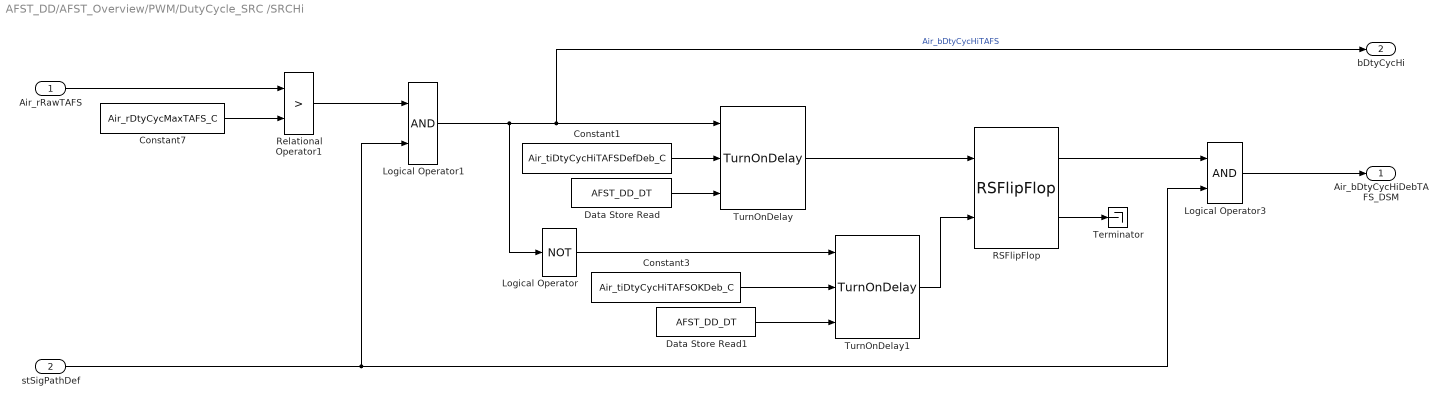
== system AFST_DD/AFST_Overview/PWM/DutyCycle_SRC /SRCHi ==
  Air_rRawTAFS : Inport
  stSigPathDef : Inport  Port=2
  Constant1 : Constant  Value=Air_tiDtyCycHiTAFSDefDeb_C
  Constant3 : Constant  Value=Air_tiDtyCycHiTAFSOKDeb_C
  Constant7 : Constant  Value=Air_rDtyCycMaxTAFS_C
  Data Store Read : DataStoreRead  DataStoreName=AFST_DD_DT
  Data Store Read1 : DataStoreRead  DataStoreName=AFST_DD_DT
  Logical Operator : Logic  Operator=NOT  AllPortsSameDT=off  OutDataTypeStr=boolean
  Logical Operator1 : Logic  AllPortsSameDT=off  OutDataTypeStr=boolean
  Logical Operator3 : Logic  AllPortsSameDT=off  OutDataTypeStr=boolean
  RSFlipFlop : CXLib/RSFlipFlop
  Relational Operator1 : RelationalOperator  Operator=>  OutDataTypeStr=boolean  RndMeth=Simplest
  Terminator : Terminator
  TurnOnDelay : CXLib/TurnOnDelay
  TurnOnDelay1 : CXLib/TurnOnDelay
  Air_bDtyCycHiDebTAFS_DSM : Outport
  bDtyCycHi : Outport  Port=2
  wires:
  Constant3/1 -> TurnOnDelay1/2
  Logical Operator1/1 -> Logical Operator/1, bDtyCycHi/1, TurnOnDelay/1  "Air_bDtyCycHiTAFS"
  Logical Operator/1 -> TurnOnDelay1/1
  Relational Operator1/1 -> Logical Operator1/1
  Constant7/1 -> Relational Operator1/2
  Data Store Read1/1 -> TurnOnDelay1/3
  Constant1/1 -> TurnOnDelay/2
  Data Store Read/1 -> TurnOnDelay/3
  RSFlipFlop/2 -> Terminator/1
  TurnOnDelay/1 -> RSFlipFlop/1
  TurnOnDelay1/1 -> RSFlipFlop/2
  Logical Operator3/1 -> Air_bDtyCycHiDebTAFS_DSM/1
  Air_rRawTAFS/1 -> Relational Operator1/1
  stSigPathDef/1 -> Logical Operator3/2, Logical Operator1/2
  RSFlipFlop/1 -> Logical Operator3/1

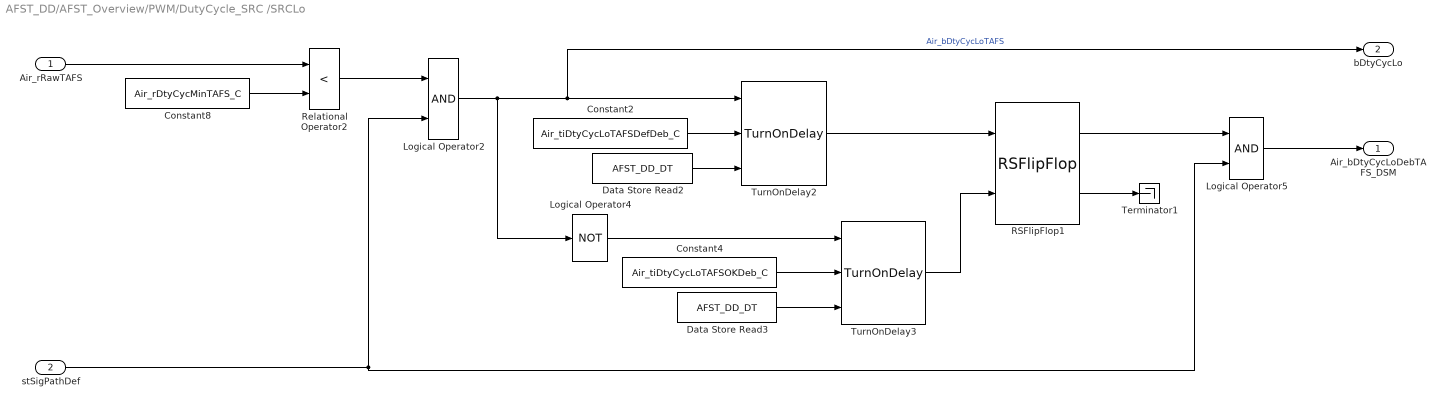
== system AFST_DD/AFST_Overview/PWM/DutyCycle_SRC /SRCLo ==
  Air_rRawTAFS : Inport
  stSigPathDef : Inport  Port=2
  Constant2 : Constant  Value=Air_tiDtyCycLoTAFSDefDeb_C
  Constant4 : Constant  Value=Air_tiDtyCycLoTAFSOKDeb_C
  Constant8 : Constant  Value=Air_rDtyCycMinTAFS_C
  Data Store Read2 : DataStoreRead  DataStoreName=AFST_DD_DT
  Data Store Read3 : DataStoreRead  DataStoreName=AFST_DD_DT
  Logical Operator2 : Logic  AllPortsSameDT=off  OutDataTypeStr=boolean
  Logical Operator4 : Logic  Operator=NOT  AllPortsSameDT=off  OutDataTypeStr=boolean
  Logical Operator5 : Logic  AllPortsSameDT=off  OutDataTypeStr=boolean
  RSFlipFlop1 : CXLib/RSFlipFlop
  Relational Operator2 : RelationalOperator  Operator=<  OutDataTypeStr=boolean  RndMeth=Simplest
  Terminator1 : Terminator
  TurnOnDelay2 : CXLib/TurnOnDelay
  TurnOnDelay3 : CXLib/TurnOnDelay
  Air_bDtyCycLoDebTAFS_DSM : Outport
  bDtyCycLo : Outport  Port=2
  wires:
  Data Store Read2/1 -> TurnOnDelay2/3
  Data Store Read3/1 -> TurnOnDelay3/3
  Constant8/1 -> Relational Operator2/2
  Relational Operator2/1 -> Logical Operator2/1
  Constant2/1 -> TurnOnDelay2/2
  Constant4/1 -> TurnOnDelay3/2
  Logical Operator4/1 -> TurnOnDelay3/1
  TurnOnDelay2/1 -> RSFlipFlop1/1
  RSFlipFlop1/1 -> Logical Operator5/1
  Logical Operator5/1 -> Air_bDtyCycLoDebTAFS_DSM/1
  RSFlipFlop1/2 -> Terminator1/1
  TurnOnDelay3/1 -> RSFlipFlop1/2
  stSigPathDef/1 -> Logical Operator5/2, Logical Operator2/2
  Logical Operator2/1 -> Logical Operator4/1, bDtyCycLo/1, TurnOnDelay2/1  "Air_bDtyCycLoTAFS"
  Air_rRawTAFS/1 -> Relational Operator2/1

== system AFST_DD/AFST_Overview/Period/Period_SRC/FinalDef ==
  Air_bPerHiDebTAFS_DSM : Inport
  Air_bPerLoDebTAFS_DSM : Inport  Port=2
  stSigPathDef : Inport  Port=3
  Logical Operator : Logic  Operator=NOT  AllPortsSameDT=off  OutDataTypeStr=boolean
  Logical Operator1 : Logic  Operator=OR  AllPortsSameDT=off  OutDataTypeStr=boolean
  Logical Operator6 : Logic  Operator=OR  AllPortsSameDT=off  OutDataTypeStr=boolean
  Air_bPerTAFSFinalDef : Outport
  wires:
  Logical Operator6/1 -> Air_bPerTAFSFinalDef/1
  Air_bPerHiDebTAFS_DSM/1 -> Logical Operator1/1
  Air_bPerLoDebTAFS_DSM/1 -> Logical Operator1/2
  Logical Operator1/1 -> Logical Operator6/1
  stSigPathDef/1 -> Logical Operator/1
  Logical Operator/1 -> Logical Operator6/2

== system AFST_DD/AFST_Overview/Period/Period_SRC/ProvDef ==
  Air_bPerTAFSFinalDef : Inport
  bDtyCycHi : Inport  Port=2
  bDtyCycLo : Inport  Port=3
  Logical Operator : Logic  Operator=OR  AllPortsSameDT=off  OutDataTypeStr=boolean
  Logical Operator1 : Logic  AllPortsSameDT=off  OutDataTypeStr=boolean
  Logical Operator2 : Logic  Operator=NOT  AllPortsSameDT=off  OutDataTypeStr=boolean
  Air_bPerTAFSProvDef : Outport
  wires:
  bDtyCycHi/1 -> Logical Operator/1
  bDtyCycLo/1 -> Logical Operator/2
  Logical Operator/1 -> Logical Operator1/1
  Air_bPerTAFSFinalDef/1 -> Logical Operator2/1
  Logical Operator2/1 -> Logical Operator1/2
  Logical Operator1/1 -> Air_bPerTAFSProvDef/1

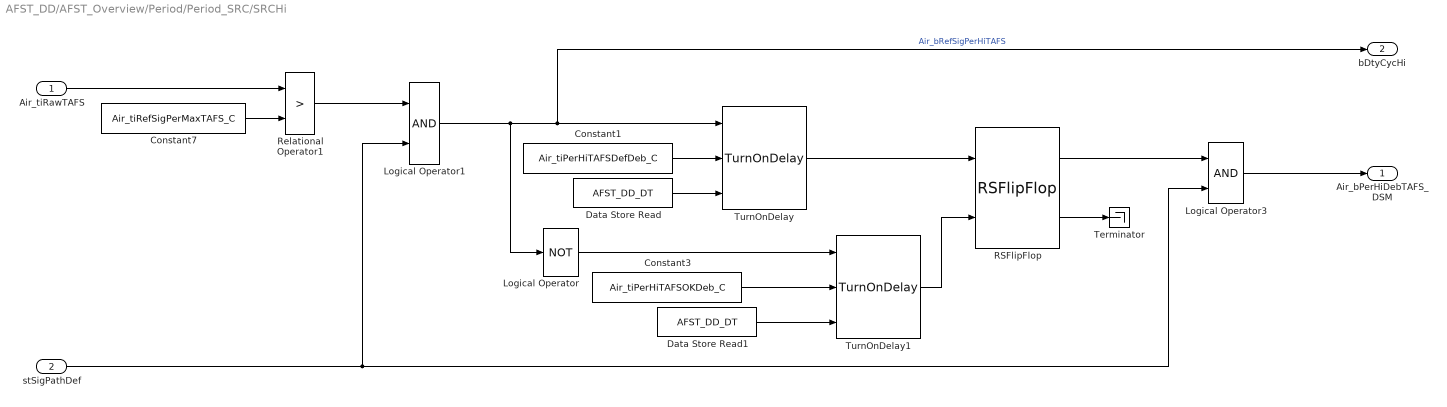
== system AFST_DD/AFST_Overview/Period/Period_SRC/SRCHi ==
  Air_tiRawTAFS : Inport
  stSigPathDef : Inport  Port=2
  Constant1 : Constant  Value=Air_tiPerHiTAFSDefDeb_C
  Constant3 : Constant  Value=Air_tiPerHiTAFSOKDeb_C
  Constant7 : Constant  Value=Air_tiRefSigPerMaxTAFS_C
  Data Store Read : DataStoreRead  DataStoreName=AFST_DD_DT
  Data Store Read1 : DataStoreRead  DataStoreName=AFST_DD_DT
  Logical Operator : Logic  Operator=NOT  AllPortsSameDT=off  OutDataTypeStr=boolean
  Logical Operator1 : Logic  AllPortsSameDT=off  OutDataTypeStr=boolean
  Logical Operator3 : Logic  AllPortsSameDT=off  OutDataTypeStr=boolean
  RSFlipFlop : CXLib/RSFlipFlop
  Relational Operator1 : RelationalOperator  Operator=>  OutDataTypeStr=boolean  RndMeth=Simplest
  Terminator : Terminator
  TurnOnDelay : CXLib/TurnOnDelay
  TurnOnDelay1 : CXLib/TurnOnDelay
  Air_bPerHiDebTAFS_DSM : Outport
  bDtyCycHi : Outport  Port=2
  wires:
  Constant3/1 -> TurnOnDelay1/2
  Logical Operator1/1 -> Logical Operator/1, bDtyCycHi/1, TurnOnDelay/1  "Air_bRefSigPerHiTAFS"
  Logical Operator/1 -> TurnOnDelay1/1
  Relational Operator1/1 -> Logical Operator1/1
  Constant7/1 -> Relational Operator1/2
  Data Store Read1/1 -> TurnOnDelay1/3
  Constant1/1 -> TurnOnDelay/2
  Data Store Read/1 -> TurnOnDelay/3
  RSFlipFlop/2 -> Terminator/1
  TurnOnDelay/1 -> RSFlipFlop/1
  TurnOnDelay1/1 -> RSFlipFlop/2
  Logical Operator3/1 -> Air_bPerHiDebTAFS_DSM/1
  Air_tiRawTAFS/1 -> Relational Operator1/1
  stSigPathDef/1 -> Logical Operator3/2, Logical Operator1/2
  RSFlipFlop/1 -> Logical Operator3/1

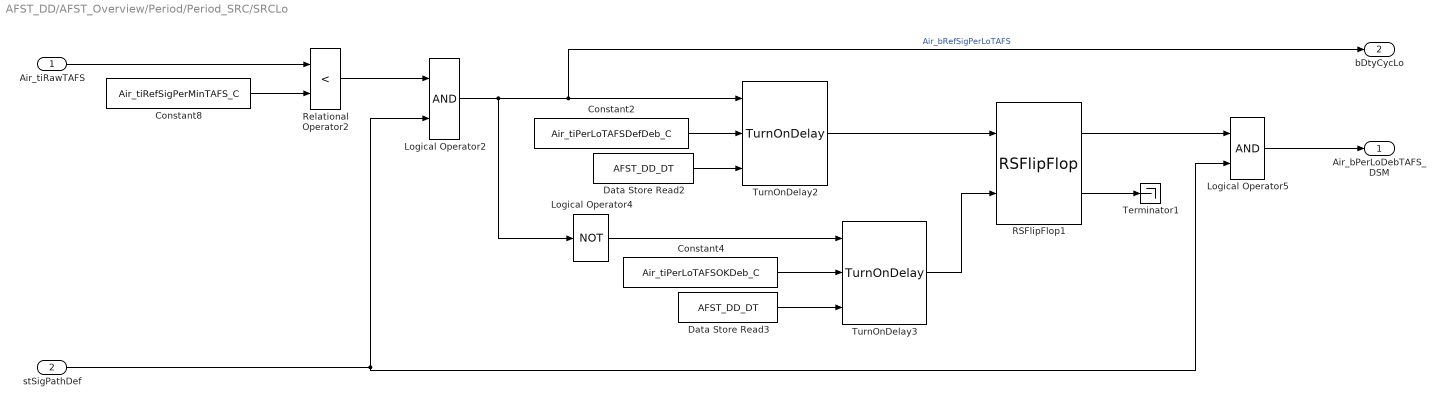
== system AFST_DD/AFST_Overview/Period/Period_SRC/SRCLo ==
  Air_tiRawTAFS : Inport
  stSigPathDef : Inport  Port=2
  Constant2 : Constant  Value=Air_tiPerLoTAFSDefDeb_C
  Constant4 : Constant  Value=Air_tiPerLoTAFSOKDeb_C
  Constant8 : Constant  Value=Air_tiRefSigPerMinTAFS_C
  Data Store Read2 : DataStoreRead  DataStoreName=AFST_DD_DT
  Data Store Read3 : DataStoreRead  DataStoreName=AFST_DD_DT
  Logical Operator2 : Logic  AllPortsSameDT=off  OutDataTypeStr=boolean
  Logical Operator4 : Logic  Operator=NOT  AllPortsSameDT=off  OutDataTypeStr=boolean
  Logical Operator5 : Logic  AllPortsSameDT=off  OutDataTypeStr=boolean
  RSFlipFlop1 : CXLib/RSFlipFlop
  Relational Operator2 : RelationalOperator  Operator=<  OutDataTypeStr=boolean  RndMeth=Simplest
  Terminator1 : Terminator
  TurnOnDelay2 : CXLib/TurnOnDelay
  TurnOnDelay3 : CXLib/TurnOnDelay
  Air_bPerLoDebTAFS_DSM : Outport
  bDtyCycLo : Outport  Port=2
  wires:
  Data Store Read2/1 -> TurnOnDelay2/3
  Data Store Read3/1 -> TurnOnDelay3/3
  Constant8/1 -> Relational Operator2/2
  Relational Operator2/1 -> Logical Operator2/1
  Constant2/1 -> TurnOnDelay2/2
  Constant4/1 -> TurnOnDelay3/2
  Logical Operator4/1 -> TurnOnDelay3/1
  TurnOnDelay2/1 -> RSFlipFlop1/1
  RSFlipFlop1/1 -> Logical Operator5/1
  Logical Operator5/1 -> Air_bPerLoDebTAFS_DSM/1
  RSFlipFlop1/2 -> Terminator1/1
  TurnOnDelay3/1 -> RSFlipFlop1/2
  stSigPathDef/1 -> Logical Operator5/2, Logical Operator2/2
  Logical Operator2/1 -> Logical Operator4/1, bDtyCycLo/1, TurnOnDelay2/1  "Air_bRefSigPerLoTAFS"
  Air_tiRawTAFS/1 -> Relational Operator2/1
